simulink model "balanced_current"  (R2015a)
settings: Solver=ode45  StartTime=0.0  StopTime=10.0  RelTol=1e-3
settings Model: Creator=rblan  LastModifiedBy=rblan

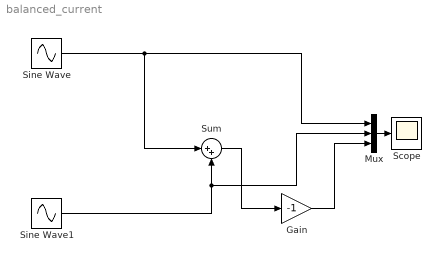
== system balanced_current ==
  Gain : Gain  Gain=-1
  Mux : Mux  Inputs=3
  Scope : Scope
  Sine Wave : Sin  SampleTime=0
  Sine Wave1 : Sin  Phase=2*pi/3  SampleTime=0
  Sum : Sum  Inputs=|++
  wires:
  Mux/1 -> Scope/1
  Sine Wave/1 -> Sum/1, Mux/1
  Sine Wave1/1 -> Mux/2, Sum/2
  Sum/1 -> Gain/1
  Gain/1 -> Mux/3
